simulink model "testrig_Linkage_Shock_HPC"  (R2024a)
settings: Solver=ode23t  StartTime=0.0  StopTime=16  RelTol=1e-3  AbsTol=1e-3  EnableMultiTasking=on
undefined symbols (not defined in the file): VDatabase
libraries: sm_lib x3, nesl_utility x2, Damper_Linear x1, fl_lib x1, simulink x1, Linkage_Shock x1, Spring_Linear x1
settings Model: Creator=smiller  LastModifiedBy=smiller
settings SolverCC: AutoScaleAbsTol=off  AlgebraicLoopSolver=TrustRegion  MaxZcPerStep=1
settings DataIOCC: LimitDataPoints=on  MaxDataPoints=10000
settings OptimizationCC: LifeSpan=inf
settings DebuggingCC: UnconnectedInputMsg=warning  UnconnectedOutputMsg=warning  UnconnectedLineMsg=warning  AllowSymbolicDim=off  SFUnexpectedBacktrackingDiag=warning  SFNoUnconditionalDefaultTransitionDiag=warning  SFExecutionAtInitializationDiag=none  ArithmeticOperatorsInVariantConditions=warning
settings ModelReferenceCC: EnableRefExpFcnMdlSchedulingChecks=on
settings SFSimCC: SimUseLocalCustomCode=off  CustomCodeUndefinedFunction=UseInterfaceOnly
settings RTWCC: RTWUseLocalCustomCode=off  GPUComputeCapability=3.5  DLArmComputeVersion=19.05
settings CodeAppCC: StateflowObjectComments=on
settings GRTTargetCC: TargetLangStandard=C89/C90 (ANSI)
settings ConfigComp: CovMetricSettings=dw  CovSaveCumulativeToWorkspaceVar=on  CovSaveSingleToWorkspaceVar=on  CovExternalEMLEnable=off  CovSFcnEnable=off
settings SimscapeCC: SimscapeLogType=all  SimscapeLogSimulationStatistics=on  SimscapeLogDataHistory=10000
settings DiagnosticsConfigSet: SimMechanicsJointTargetOverSpecification=warning
settings ExplorerConfigSet: InternalSimMechanicsExplorerSettings="<ExplorerConfiguration><canonicalview>default</canonicalview><AnimationSetting><BasePlaybackSpeed>1.0</BasePlaybackSpeed><PlaybackSpeedFactor>1.0</PlaybackSpeedFactor></AnimationSetting><TilePanel><TileInfo><Tiles Columns=\"1\" Count=\"1\" Rows=\"1\"><Column Weight=\"1\"/><Row Weight=\"1\"/><Tile Height=\"1\" Width=\"1\" X=\"0\" Y=\"0\"/></Tiles></TileInfo><SceneInfo><SceneViewer><BGColor><R>1</R><G>1</G><B>1</B></BGColor><Camera><DoPerspective>off</DoPerspective><Position><X>0.999999970860395493</X><Y>5.51556356143123594e-10</Y><Z>0.0619756028561508493</Z></Position><Center><X>-2.91396045071223853e-08</X><Y>5.51556356143123594e-10</Y><Z>0.0619756028561508493</Z></Center><Up><X>-0</X><Y>0</Y><Z>1</Z></Up><ViewLimDist>1</ViewLimDist><YLim>0.214265129417181011</YLim><XLim>0.295786878993414826</XLim></Camera></SceneViewer></SceneInfo></TilePanel><MechEditorPanel><Cameras/><GfxPanelCameraMap/><VideoCreator><PlaybackSpeedRatio>1.0</PlaybackSpeedRatio><FrameRate>30</FrameRate><VideoFormat>Motion JPEG AVI</VideoFormat><FrameSize>auto</FrameSize></VideoCreator></MechEditorPanel></ExplorerConfiguration>"

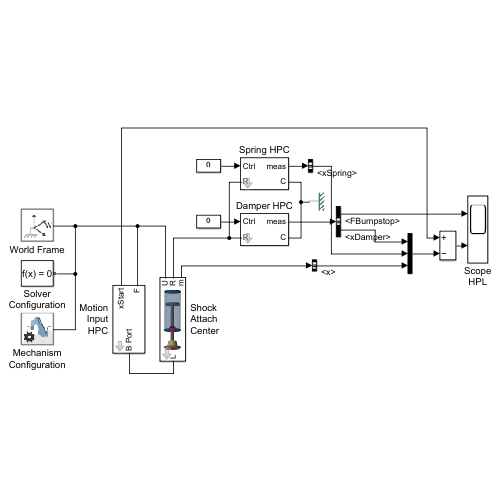
[thumbnail: Simulink's stored preview of the top-level diagram]
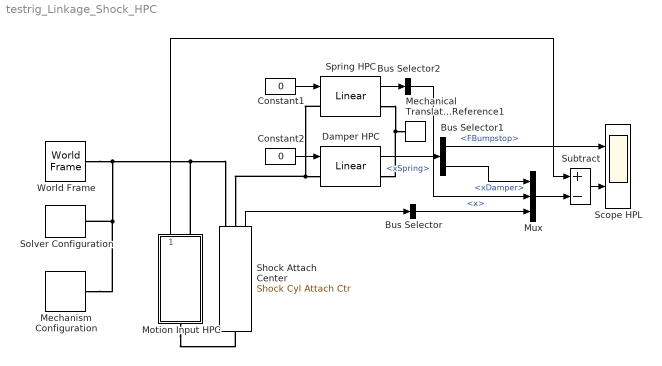
== system testrig_Linkage_Shock_HPC ==
  Bus Selector : BusSelector  OutputSignals=x
  Bus Selector1 : BusSelector  OutputSignals=FBumpstop,xDamper
  Bus Selector2 : BusSelector  OutputSignals=xSpring
  Constant1 : Constant  Value=0
  Constant2 : Constant  Value=0
  Damper HPC : Damper_Linear/Linear  VariantControl=Linear  dam_b=VDatabase.Damper.SUV_Landy_TA2PR_AsymmetricLinear_A1.Damping.d.Value  hp_dpr_top=VDatabase.Damper.SUV_Landy_TA2PR_AsymmetricLinear_A1.Damping.sTopL.Value  hp_dpr_bot=VDatabase.Damper.SUV_Landy_TA2PR_AsymmetricLinear_A1.Damping.sBottomL.Value  bs_lim_upper=VDatabase.Damper.SUV_Landy_TA2PR_AsymmetricLinear_A1.Endstop.xMax.Value  bs_lim_lower=VDatabase.Damper.SUV_Landy_TA2PR_AsymmetricLinear_A1.Endstop.xMin.Value  bs_k_upper=VDatabase.Damper.SUV_Landy_TA2PR_AsymmetricLinear_A1.Endstop.KxMax.Value  bs_k_lower=VDatabase.Damper.SUV_Landy_TA2PR_AsymmetricLinear_A1.Endstop.KxMin.Value  bs_b_upper=VDatabase.Damper.SUV_Landy_TA2PR_AsymmetricLinear_A1.Endstop.dxMax.Value  bs_b_lower=VDatabase.Damper.SUV_Landy_TA2PR_AsymmetricLinear_A1.Endstop.dxMin.Value  bs_region=VDatabase.Damper.SUV_Landy_TA2PR_AsymmetricLinear_A1.Endstop.xTransition.Value
  Mechanical Translational Reference1 : fl_lib/Mechanical/Translational Elements/Mechanical Translational Reference
  Mechanism Configuration : sm_lib/Utilities/Mechanism Configuration  UniformGravity=Constant  GravityVector=[0 0 -9.80665]  GravityVectorUnits=m/s^2  LinearizationDelta=0.001  JointModeTransitionNonlinearIterations=2
  Motion Input HPC : Subsystem  mask{hp_top=VDatabase.Susp.AxleTA2PR_SUV_Landy_f.AxleTA2PR.Shock.sTopL.Value, hp_bot=VDatabase.Susp.AxleTA2PR_SUV_Landy_f.AxleTA2PR.Shock.sBottomL.Value, xMax=VDatabase.Susp.AxleTA2PR_SUV_Landy_f.AxleTA2PR.Endstop.xMax.Value, xMin=VDatabase.Susp.AxleTA2PR_SUV_Landy_f.AxleTA2PR.Endstop.xMin.Value, xPen=1e-3}
      mask prompts: hp_top "HP Top"; hp_bot "HP Bottom"; xMax "Upper Lim"; xMin "Lower Lim"; xPen "Penetration"
      mask init:
      | xStart = sqrt(sum((hp_top-hp_bot).^2));
  Mux : Mux  Inputs=3
  Scope HPL : Scope  NumInputPorts=2
  Shock Attach Center : Linkage_Shock/Shock Cyl Attach Ctr  shock_pist_mass=VDatabase.Susp.AxleTA2PR_SUV_Landy_f.AxleTA2PR.Shock.mPiston.Value  shock_cyl_mass=VDatabase.Susp.AxleTA2PR_SUV_Landy_f.AxleTA2PR.Shock.mCylinder.Value  hp_spr_top=VDatabase.Susp.AxleTA2PR_SUV_Landy_f.AxleTA2PR.Shock.sTopL.Value  hp_spr_bot=VDatabase.Susp.AxleTA2PR_SUV_Landy_f.AxleTA2PR.Shock.sBottomL.Value  up_lim_bumpstop=VDatabase.Susp.AxleTA2PR_SUV_Landy_f.AxleTA2PR.Endstop.xMax.Value  low_lim_bumpstop=VDatabase.Susp.AxleTA2PR_SUV_Landy_f.AxleTA2PR.Endstop.xMin.Value  clr_conn_shock=Visual.hp.clr  opc_conn_shock=Visual.hp.opc  size_conn_shock=Visual.hp.rad  clr_shock_cyl=Visual.clr.blue  opc_shock_cyl=Visual.part.opc  radius_shock_cyl=0.05  clr_shock_piston=Visual.clr.gray  opc_shock_piston=Visual.part.opc  clr_shock_bumpstop=Visual.clr.yellowpale  opc_shock_bumpstop=Visual.part.opc  deadvol_len_shock_cyl=Visual.Shock.dead_length  piston_len_shock=Visual.Shock.piston.len  cyl_cap_len_shock=Visual.Shock.cap.len  bumpstop_len_shock=Visual.Shock.bumpstop.len
  Solver Configuration : nesl_utility/Solver Configuration  PhysicalDomain=network_engine_domain  SubClassName=solver  LeftPortType=input  RightPortType=generic  Tones=[]  Harmonics=[]  SimulateNoise=off  Profile=off  UseLocalSampling=off  EnableSwitchedLinearOptims=on  FrequencyDomain=off  UseCCode=off  RelTol=0.001  AbsTol=1e-06  MinStep=1e-09  ToWorkspace=off  RevertToSquareIcSolve=off  NumHomotopyIterations=100  PhasorMode=off  PhasorModeNumHarmonics=1  ConsistencySolver=NEWTON_FTOL  IndexReductionMethod=DerivativeReplacement  DoDC=off  ResidualTolerance=1e-09  ConsistencyTolSource=GLOBAL  ConsistencyAbsTol=0.001  ConsistencyRelTol=0.001  ConsistencyTolFactor=0.001  UseLocalSolver=off  LocalSolverChoice=NE_BACKWARD_EULER_ADVANCER  ResolveIndetEquations=on  FunctionEvalNumThread=1  LocalSolverSampleTime=0.001  DoFixedCost=off  MaxNonlinIter=3  MaxModeIter=2  ComputeImpulses=off  ImpulseIterations=2  LinearAlgebra=Sparse  LinearAlgebraNumThread=0  EquationFormulation=NE_TIME_EF  DelaysMemoryBudget=1024  AutomaticFiltering=on  FilteringTimeConstant=0.001  PartitionStorageMethod=AS_NEEDED  PartitionMemoryBudget=1024  PartitionMethod=FAST  MultibodyUseLocalSolver=off  MultibodyLocalSolverChoice=ODE1  MultibodyLocalSolverSampleTime=0.001
  Spring HPC : Spring_Linear/Linear  VariantControl=Linear  spr_def0=VDatabase.Spring.SUV_Landy_TA2PR_AsymmetricLinear_A1.xPreloadL.Value  spr_frc0=VDatabase.Spring.SUV_Landy_TA2PR_AsymmetricLinear_A1.fPreloadL.Value  spr_k=VDatabase.Spring.SUV_Landy_TA2PR_AsymmetricLinear_A1.K.Value  spr_hp_top=VDatabase.Spring.SUV_Landy_TA2PR_AsymmetricLinear_A1.sTopL.Value  spr_hp_bot=VDatabase.Spring.SUV_Landy_TA2PR_AsymmetricLinear_A1.sBottomL.Value
  Subtract : Sum  Inputs=+-
  World Frame : sm_lib/Frames and Transforms/World Frame
  wires:
  Spring HPC/1 -> Bus Selector2/1
  Constant1/1 -> Spring HPC/1
  Shock Attach Center/1 -> Bus Selector/1
  Constant2/1 -> Damper HPC/1
  Damper HPC/1 -> Bus Selector1/1
  Bus Selector1/1 -> Scope HPL/1  "<FBumpstop>"
  Bus Selector/1 -> Mux/3  "<x>"
  Bus Selector1/2 -> Mux/1  "<xDamper>"
  Mux/1 -> Subtract/2
  Bus Selector2/1 -> Mux/2  "<xSpring>"
  Motion Input HPC/1(xStart) -> Subtract/1
  Subtract/1 -> Scope HPL/2
  connections:
  Spring HPC/LConn1 -- Shock Attach Center/RConn1 -- Damper HPC/LConn1
  Spring HPC/RConn1 -- Damper HPC/RConn1 -- Mechanical Translational Reference1/LConn1
  Mechanism Configuration/RConn1 -- World Frame/RConn1 -- Motion Input HPC/RConn1 -- Shock Attach Center/RConn2 -- Solver Configuration/RConn1
  Motion Input HPC/LConn1 -- Shock Attach Center/LConn1

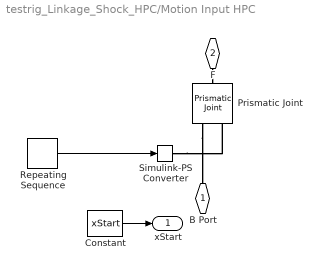
== system testrig_Linkage_Shock_HPC/Motion Input HPC ==
  Constant : Constant  Value=xStart
  Prismatic Joint : sm_lib/Joints/Prismatic Joint  JointMode=Normal  CompositeWrenchDir=FollowerOnBase  CompositeWrenchFrame=BaseFrame  SenseConstraintForce=off  SenseConstraintTorque=off  SenseTotalForce=off  SenseTotalTorque=off  PositionTargetSpecify=on  PositionTargetPriority=High  PositionTargetValue=xStart  PositionTargetValueUnits=m  VelocityTargetSpecify=off  VelocityTargetPriority=High  VelocityTargetValue=0  VelocityTargetValueUnits=m/s  EquilibriumPosition=0  EquilibriumPositionUnits=m  SpringStiffness=0  SpringStiffnessUnits=N/m  DampingCoefficient=0  DampingCoefficientUnits=N/(m/s)  LowerLimitSpecify=off  LowerLimitBound=-1  LowerLimitBoundUnits=m  LowerLimitStiffness=1e6  LowerLimitStiffnessUnits=N/m  LowerLimitDamping=1e3  LowerLimitDampingUnits=N/(m/s)  LowerLimitTransitionRegionWidth=1e-4  LowerLimitTransitionRegionWidthUnits=m  UpperLimitSpecify=off  UpperLimitBound=1  UpperLimitBoundUnits=m  UpperLimitStiffness=1e6  UpperLimitStiffnessUnits=N/m  UpperLimitDamping=1e3  UpperLimitDampingUnits=N/(m/s)  UpperLimitTransitionRegionWidth=1e-4  UpperLimitTransitionRegionWidthUnits=m  TorqueActuationMode=ComputedTorque  MotionActuationMode=InputMotion  SensePosition=off  SenseVelocity=off  SenseAcceleration=off  SenseTorqueForce=off  SenseLowerLimitTorqueForce=off  SenseUpperLimitTorqueForce=off
  Repeating Sequence : simulink/Sources/Repeating Sequence  rep_seq_t=[0 2 4 6 8 10 12 14 16]  rep_seq_y=[0 0 xMax xMax+xPen 0 xMin xMin-xPen 0 0]+xStart
  Simulink-PS Converter : nesl_utility/Simulink-PS Converter  PhysicalDomain=network_engine_domain  SubClassName=ps_input  LeftPortType=input  RightPortType=output  PseudoPeriodic=off  Frequencies=[]  NoiseDistribution=none  NoiseParameters=[]  Unit=m  AffineConversion=off  FilteringAndDerivatives=filter  SimscapeFilterOrder=2  InputFilterTimeConstant=0.1  UdotUserProvided=0
  B Port : PMIOPort  Side=Left
  F : PMIOPort  Port=2  Side=Right
  xStart : Outport
  wires:
  Repeating Sequence/1 -> Simulink-PS Converter/1
  Constant/1 -> xStart/1
  connections:
  Simulink-PS Converter/RConn1 -- Prismatic Joint/LConn2
  Prismatic Joint/LConn1 -- B Port/RConn1
  F/RConn1 -- Prismatic Joint/RConn1
